simulink model "Engranajes (1)"  (R2015a)
settings: Solver=ode45  StartTime=0.0  StopTime=10.0  RelTol=1e-3
undefined symbols (not defined in the file): magnitude
libraries: simulink x2
settings Model: Creator=Henry Alberto  LastModifiedBy=Henry Alberto

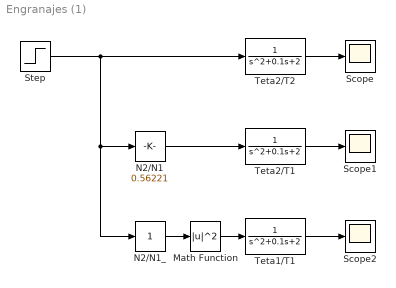
== system Engranajes (1) ==
  Math Function : Math  Operator=magnitude^2  SaturateOnIntegerOverflow=on
  N2/N1 : simulink/Math Operations/Slider Gain  low=0  gain=0.56221  high=2
  N2/N1_ : simulink/Math Operations/Slider Gain  low=0  gain=1  high=2
  Scope : Scope
  Scope1 : Scope
  Scope2 : Scope
      settings: SaveName=ScopeData2
  Step : Step  SampleTime=0
  Teta1/T1 : TransferFcn  Denominator=[1 0.1 2]
  Teta2/T1 : TransferFcn  Denominator=[1 0.1 2]
  Teta2/T2 : TransferFcn  Denominator=[1 0.1 2]
  wires:
  Step/1 -> N2/N1_/1, N2/N1/1, Teta2/T2/1
  Teta2/T2/1 -> Scope/1
  N2/N1/1 -> Teta2/T1/1
  N2/N1_/1 -> Math Function/1
  Math Function/1 -> Teta1/T1/1
  Teta2/T1/1 -> Scope1/1
  Teta1/T1/1 -> Scope2/1
